simulink model "speedController"  (R2025b)
settings: Solver=FixedStepDiscrete  StartTime=0.0  StopTime=10.0  FixedStep=1e-3  RelTol=1e-3
undefined symbols (not defined in the file or in its folder): controller_mode, controller_modes, controllerGains
libraries: simulink_extras x2, simulink x1, metux_library x1
settings Model: DataDictionary=pid.sldd  Creator=karadeli  LastModifiedBy=karadeli
settings OptimizationCC: DefaultParameterBehavior=Inlined  GainParamInheritBuiltInType=on  UseFloatMulNetSlope=on  InlineInvariantSignals=on  PassReuseOutputArgsAs=Individual arguments  ZeroExternalMemoryAtStartup=off  ZeroInternalMemoryAtStartup=off  NoFixptDivByZeroProtection=on  EfficientFloat2IntCast=on  LifeSpan=1  OptimizeBlockOrder=speed  DifferentSizesBufferReuse=on  EfficientTunableParamExpr=on
settings DebuggingCC: ParamSuppressDoubleToSinglePrecisionLossMsg=on  ParameterTunabilityLossMsg=none
settings HardwareCC: ProdBitPerPointer=32.0  ProdBitPerSizeT=32.0  ProdBitPerPtrDiffT=32.0  ProdLargestAtomicInteger=Long  ProdLargestAtomicFloat=Double  ProdWordSize=32.0  ProdLongLongMode=on  ProdHWDeviceType=ARM Compatible->ARM Cortex-M
settings SFSimCC: MATLABDynamicMemAlloc=off
settings RTWCC: SystemTargetFile=ert.tlc  GenCodeOnly=on  TemplateMakefile=ert_default_tmf  TargetLang=C++  Description=Embedded Coder
settings CodeAppCC: ForceParamTrailComments=on  IgnoreCustomStorageClasses=off  OperatorAnnotations=on  SimulinkDataObjDesc=on  SFDataObjDesc=on  CustomSymbolStrGlobalVar=rt$N$M  CustomSymbolStrType=$N$M  CustomSymbolStrFcn=$N$M$F  CustomSymbolStrMacro=$N$M  InsertBlockDesc=on
settings ERTTargetCC: RootIOFormat=Structure reference  ERTCustomFileTemplate=example_file_process.tlc  ERTFilePackagingFormat=CompactWithDataFile  TargetLangStandard=C++11 (ISO)  GenerateSampleERTMain=on  IncludeMdlTerminateFcn=off  CombineSignalStateStructs=on  SuppressErrorStatus=on  SupportAbsoluteTime=off  CodeInterfacePackaging=C++ class  SubcomponentCodeInterfacePackaging=C++ class  SupportComplex=off

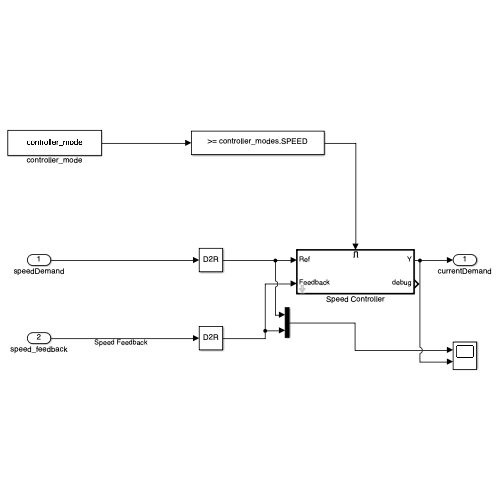
[thumbnail: Simulink's stored preview of the top-level diagram]
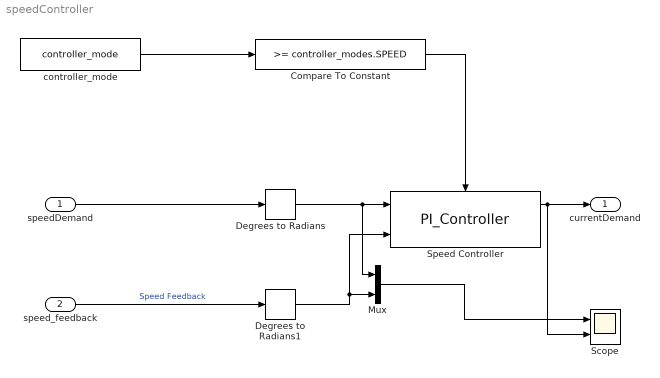
== system speedController ==
  speedDemand : Inport  Unit=deg/s
  speed_feedback : Inport  Port=2  Unit=deg/s  SampleTime=controllerGains.speed.Ts  Interpolate=off
  Compare To Constant : simulink/Logic and Bit Operations/Compare To Constant  relop=>=  const=controller_modes.SPEED  OutDataTypeStr=boolean
  Degrees to Radians : simulink_extras/Transformations/Degrees to Radians
  Degrees to Radians1 : simulink_extras/Transformations/Degrees to Radians
  Mux : Mux  Inputs=2
  Scope : Scope  NumInputPorts=2
      settings: ActiveDisplayYMinimum=-3482.2818450927725  ActiveDisplayYMaximum=28164.697982788086
  Speed Controller : metux_library/PI_Controller  Kp=controllerGains.speed.Kp  Ki=controllerGains.speed.Ki  SatMax=controllerGains.speed.SatMax  SatMin=controllerGains.speed.SatMin  Ts=controllerGains.speed.Ts  RateLimiterMax=controllerGains.speed.RateLimiterMax  RateLimiterMin=controllerGains.speed.RateLimiterMin
  controller_mode : Constant  Value=controller_mode  SampleTime=-1
  currentDemand : Outport  Unit=A
  wires:
  Compare To Constant/1 -> Speed Controller/Enable
  controller_mode/1 -> Compare To Constant/1
  speed_feedback/1 -> Degrees to Radians1/1  "Speed Feedback"
  Degrees to Radians/1 -> Mux/1, Speed Controller/1
  speedDemand/1 -> Degrees to Radians/1
  Degrees to Radians1/1 -> Speed Controller/2, Mux/2
  Speed Controller/1 -> currentDemand/1, Scope/2
  Mux/1 -> Scope/1
